simulink model "TrafficLightSystem_MooreSemantic"  (R2020a)
settings: Solver=VariableStepAuto  StartTime=0.0  StopTime=200  RelTol=1e-3
undefined symbols (not defined in the file): DiscIntNeverNeededParam
libraries: simulink x1
settings Model: Creator=DELL  LastModifiedBy=DELL

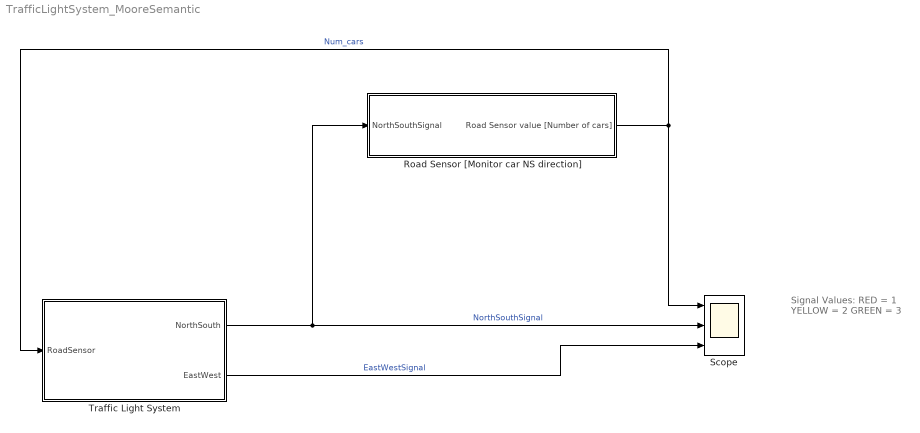
== system TrafficLightSystem_MooreSemantic ==
  note: Signal Values:
      | RED = 1
      | YELLOW = 2
      | GREEN = 3
  Road Sensor [Monitor car NS direction] : Subsystem
  Scope : Scope  NumInputPorts=3
  Traffic Light System : Stateflow chart  TreatAsAtomicUnit=on
  wires:
  Traffic Light System/1(NorthSouth) -> Road Sensor [Monitor car NS direction]/1(NorthSouthSignal), Scope/2  "NorthSouthSignal"
  Road Sensor [Monitor car NS direction]/1(Road Sensor value [Number of cars]) -> Traffic Light System/1(RoadSensor), Scope/1  "Num_cars"
  Traffic Light System/2(EastWest) -> Scope/3  "EastWestSignal"

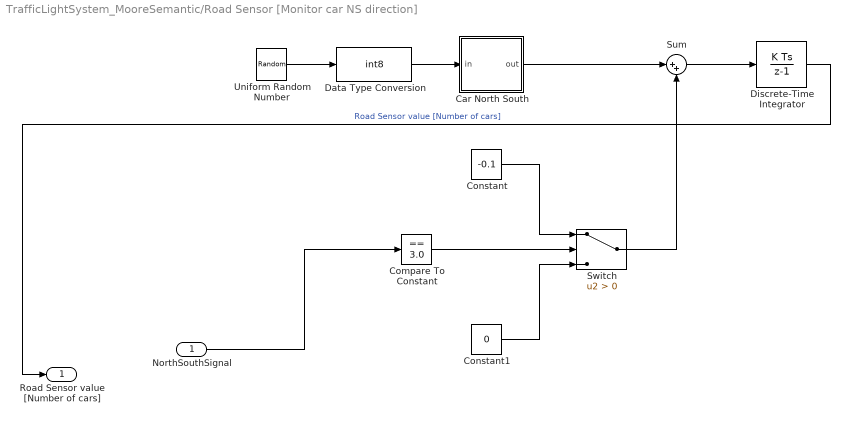
== system TrafficLightSystem_MooreSemantic/Road Sensor [Monitor car NS direction] ==
  NorthSouthSignal : Inport
  Car North South : Stateflow chart  TreatAsAtomicUnit=on
  Compare To Constant : simulink/Logic and Bit Operations/Compare To Constant  relop===  const=3.0  OutDataTypeStr=boolean
  Constant : Constant  Value=-0.1
  Constant1 : Constant  Value=0
  Data Type Conversion : DataTypeConversion  OutDataTypeStr=int8
  Discrete-Time Integrator : DiscreteIntegrator  SampleTime=-1  LimitOutput=on  LowerSaturationLimit=0  ICPrevOutput=DiscIntNeverNeededParam  ICPrevScaledInput=DiscIntNeverNeededParam
  Sum : Sum  Inputs=|++
  Switch : Switch  Criteria=u2 > Threshold
  Uniform Random Number : UniformRandomNumber  Minimum=0  Maximum=100  SampleTime=0.1
  Road Sensor value [Number of cars] : Outport
  wires:
  NorthSouthSignal/1 -> Compare To Constant/1
  Constant/1 -> Switch/1
  Compare To Constant/1 -> Switch/2
  Uniform Random Number/1 -> Data Type Conversion/1
  Discrete-Time Integrator/1 -> Road Sensor value [Number of cars]/1  "Road Sensor value [Number of cars]"
  Switch/1 -> Sum/2
  Data Type Conversion/1 -> Car North South/1(in)
  Sum/1 -> Discrete-Time Integrator/1
  Car North South/1(out) -> Sum/1
  Constant1/1 -> Switch/3

== stateflow chart TrafficLightSystem_MooreSemantic/Road Sensor [Monitor car NS direction]/Car North South ==
  (default) -> (junction 1) : {out = in > 98;}
  data: out output; in input

== stateflow chart TrafficLightSystem_MooreSemantic/Traffic Light System ==
  state NorthSouthStop
    NorthSouth = RED;
    EastWest = GREEN;
  state NorthSouthCheck
    NorthSouth = RED;
    EastWest = GREEN;
  state NorthSouthStopTOGo
    NorthSouth = RED;
    EastWest = YELLOW;
  state EastWestStopToGo
    NorthSouth = YELLOW;
    EastWest = RED;
  state NorthSouthGo
    NorthSouth = GREEN;
    EastWest = RED;
  (default) -> NorthSouthStop
  NorthSouthStop -> NorthSouthCheck : after(20,tick)
  NorthSouthCheck -> NorthSouthStopTOGo : [RoadSensor]
  EastWestStopToGo -> NorthSouthStop : after(3,tick)
  NorthSouthStopTOGo -> NorthSouthGo : after(3,tick)
  NorthSouthGo -> EastWestStopToGo : after(10,tick)
  data: NorthSouth output; RED constant double =1; YELLOW constant double =2; GREEN constant double =3; EastWest output; RoadSensor input
